simulink model "Accelerometer"  (R2022b)
settings: Solver=VariableStepAuto  StartTime=0.0  StopTime=10.0  RelTol=1e-3
libraries: aerolibnav x1
settings Model: Creator=Fabian  LastModifiedBy=Fabian

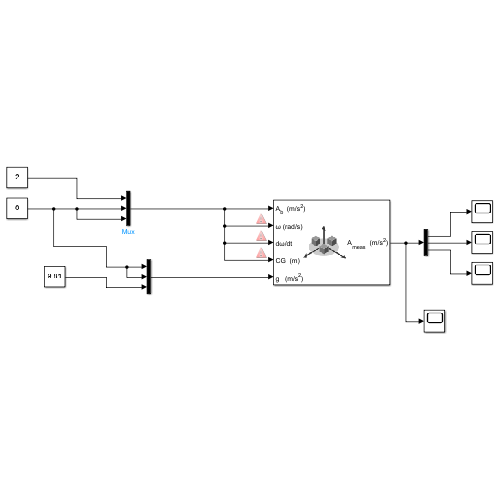
[thumbnail: Simulink's stored preview of the top-level diagram]
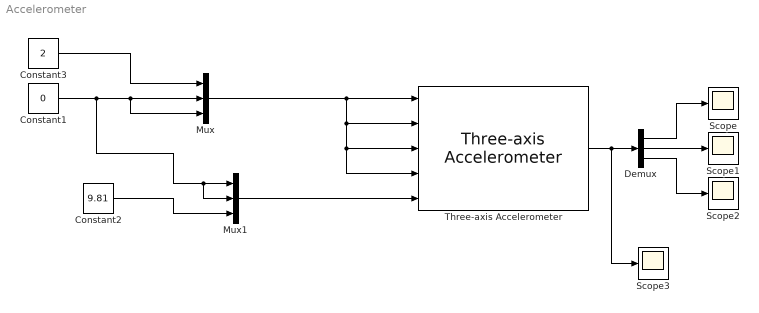
== system Accelerometer ==
  Constant1 : Constant  Value=0
  Constant2 : Constant  Value=9.81
  Constant3 : Constant  Value=2
  Demux : Demux  Outputs=3
  Mux : Mux  Inputs=3
  Mux1 : Mux  Inputs=3
  Scope{,1..3} (4 alike) : Scope
  Three-axis Accelerometer : aerolibnav/Three-axis Accelerometer  units=Metric (MKS)  acc=[0 0 0]  gtype=on  dtype_a=on  w_a=190  z_a=0.707  a_sf_cc=[1 0 0; 0 1 0; 0 0 1]  a_bias=[0 0 0]  a_Ts=0  a_rand=off  a_seeds=[23093 23094 23095]  a_pow=[0.001 0.001 0.001]  a_sat="[-inf  -inf  -inf  inf inf inf]"
  wires:
  Constant1/1 -> Mux1/2, Mux1/1, Mux/3, Mux/2
  Mux/1 -> Three-axis Accelerometer/4, Three-axis Accelerometer/3, Three-axis Accelerometer/2, Three-axis Accelerometer/1
  Constant2/1 -> Mux1/3
  Mux1/1 -> Three-axis Accelerometer/5
  Three-axis Accelerometer/1 -> Scope3/1, Demux/1
  Demux/3 -> Scope2/1
  Demux/2 -> Scope1/1
  Demux/1 -> Scope/1
  Constant3/1 -> Mux/1
